simulink model "P2_Q3"  (R2023a)
settings: Solver=VariableStepAuto  StartTime=0.0  StopTime=52  RelTol=1e-3
settings Model: Creator=asus  LastModifiedBy=asus

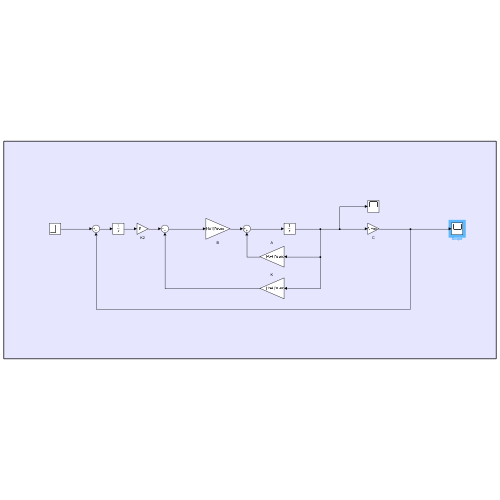
[thumbnail: Simulink's stored preview of the top-level diagram]
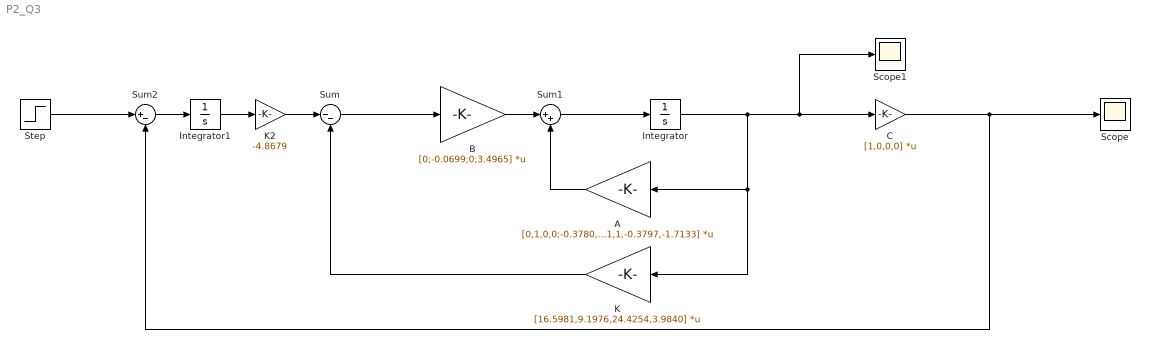
== system P2_Q3 ==
  A : Gain  Gain=[0,1,0,0;-0.3780,0,7.0147,0.0343;0,0,0,1;18.9001,1,-0.3797,-1.7133]  Multiplication=Matrix(K*u) (u vector)
  B : Gain  Gain=[0;-0.0699;0;3.4965]  Multiplication=Matrix(K*u) (u vector)
  C : Gain  Gain=[1,0,0,0]  Multiplication=Matrix(K*u) (u vector)
  Integrator : Integrator
  Integrator1 : Integrator
  K : Gain  Gain=[16.5981,9.1976,24.4254,3.9840]  Multiplication=Matrix(K*u) (u vector)
  K2 : Gain  Gain=-4.8679
  Scope : Scope
  Scope1 : Scope
  Step : Step  Time=0  After=0.1  SampleTime=0
  Sum : Sum  Inputs=|--
  Sum1 : Sum  Inputs=|++
  Sum2 : Sum  Inputs=|+-
  wires:
  K/1 -> Sum/2
  A/1 -> Sum1/2
  B/1 -> Sum1/1
  C/1 -> Scope/1, Sum2/2
  K2/1 -> Sum/1
  Sum1/1 -> Integrator/1
  Sum2/1 -> Integrator1/1
  Integrator/1 -> K/1, A/1, C/1, Scope1/1
  Step/1 -> Sum2/1
  Sum/1 -> B/1
  Integrator1/1 -> K2/1
